simulink model "Proj3_PMSM_ForStudent"  (Simulink 8.0)
settings: Solver=ode45  StartTime=0.0  StopTime=0.5  MaxStep=1e-5  RelTol=1e-3
InitFcn:
  | Idc=0;
  | Vabc=0;
  | Iw=0;
values from neighbouring files (symbols this model uses):
  Flux = 0.7213*BaseFlux    [MSE452_Lab3_parameters.m]
  Ld = 0.7029*Lb    [MSE452_Lab3_parameters.m]
  Lq = 0.7029*Lb    [MSE452_Lab3_parameters.m]
  OMEGAb_r = OMEGAb/Ppairs    (= 41.885284054)    [MSE452_Lab3_parameters.m]
  Ppairs = 8    [MSE452_Lab3_parameters.m]
  Rs = 0.00517*Zb    [MSE452_Lab3_parameters.m]
undefined symbols (not defined in the file or in its folder): Ts
libraries: powerlib x1
settings Model: Creator=Administrator  LastModifiedBy=dw  BufferReuse=off
settings SolverCC: ZeroCrossControl=DisableAll
settings DataIOCC: SignalLoggingSaveFormat=ModelDataLogs
settings OptimizationCC: BlockReduction=off  InlineParams=on  BufferReuse=off  InitFltsAndDblsToZero=on
settings DebuggingCC: SaveWithParameterizedLinksMsg=none  SignalResolutionControl=TryResolveAllWithWarning  MultiTaskDSMMsg=warning  MultiTaskCondExecSysMsg=none  FcnCallInpInsideContextMsg=UseLocalSettings  StrictBusMsg=Warning
settings RTWCC: IncludeERTFirstTime=on
settings GRTTargetCC: TargetFcnLib=ansi_tfl_tmw.mat  CombineOutputUpdateFcns=off  GRTInterface=on

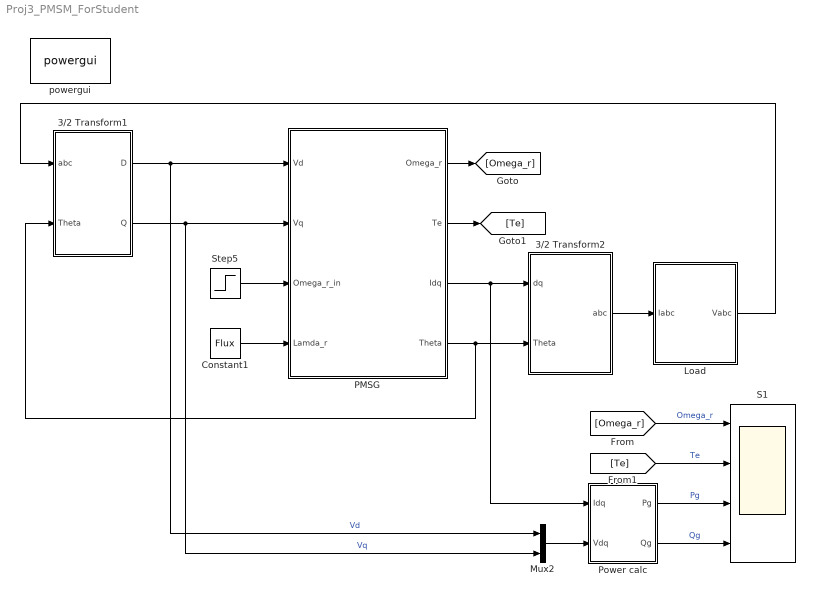
== system Proj3_PMSM_ForStudent ==
  3/2 Transform1 : Subsystem
  3/2 Transform2 : Subsystem
  Constant1 : Constant  Value=Flux
  Load : Subsystem
  Mux2 : Mux  Inputs=2
  PMSG : Subsystem
  Power calc : Subsystem
  S1 : Scope  NumInputPorts=4
      settings: TimeRange=1  YMin=-500~-30~120~1750  YMax=3500~50~210~3500  SaveName=SpeedTorquePower
  Step5 : Step  Time=0  After=1.0*OMEGAb_r  SampleTime=0
  powergui : powerlib/powergui  SimulationMode=Continuous  SolverType=Tustin  SampleTime=Ts  frequency=60  SPID=off  DisableSnubberDevices=off  DisableRonSwitches=off  DisableVfSwitches=off  SwTol=0  Interpol=off  DisplayEquations=off  FunctionMessages=off  frequencyindice=1  Pbase=100e6  ErrMax=1e-4  Iterations=50  UnitsV=kV  UnitsW=MW  echomessages=off  HookPort=off  EnableUseOfTLC=off  x0status=blocks  RestoreLinks=warning  ResistiveCurrentMeasurement=off  Frange=[0:2:500]  Ylog=off  Xlog=on  ShowGrid=off  save=off  variable=ZData  structure=GridVIWave  ZoomFFT=off  StartTime=2  cycles=12  DisplayStyle=1  fundamental=60  FreqAxis=on  MaxFrequency=60*15  frequencyindicesteady=1  RmsSteady=1  display=off  Ts=0  methode=off
  wires:
  PMSG/3(Idq) -> 3/2 Transform2/1(dq), Power calc/1(Idq)
  3/2 Transform1/2(Q) -> PMSG/2(Vq), Mux2/2  "Vq"
  3/2 Transform1/1(D) -> PMSG/1(Vd), Mux2/1  "Vd"
  PMSG/1(Omega_r) -> [Omega_r]
  PMSG/2(Te) -> [Te]
  Step5/1 -> PMSG/3(Omega_r_in)
  PMSG/4(Theta) -> 3/2 Transform2/2(Theta), 3/2 Transform1/2(Theta)
  Mux2/1 -> Power calc/2(Vdq)
  Constant1/1 -> PMSG/4(Lamda_r)
  3/2 Transform2/1(abc) -> Load/1(Iabc)
  Load/1(Vabc) -> 3/2 Transform1/1(abc)
  Power calc/2(Qg) -> S1/4  "Qg"
  Power calc/1(Pg) -> S1/3  "Pg"
  [Omega_r] -> S1/1  "Omega_r"
  [Te] -> S1/2  "Te"

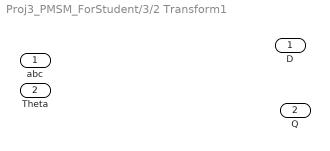
== system Proj3_PMSM_ForStudent/3/2 Transform1 ==
  abc : Inport
  Theta : Inport  Port=2
  D : Outport
  Q : Outport  Port=2

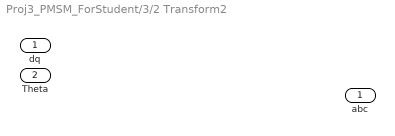
== system Proj3_PMSM_ForStudent/3/2 Transform2 ==
  dq : Inport
  Theta : Inport  Port=2
  abc : Outport

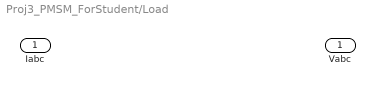
== system Proj3_PMSM_ForStudent/Load ==
  Iabc : Inport
  Vabc : Outport

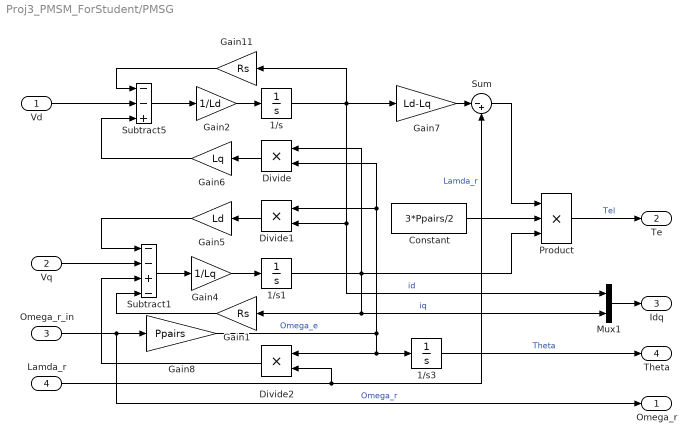
== system Proj3_PMSM_ForStudent/PMSG ==
  Vd : Inport
  Vq : Inport  Port=2
  Omega_r_in : Inport  Port=3
  Lamda_r : Inport  Port=4
  1/s : Integrator
  1/s1 : Integrator
  1/s3 : Integrator
  Constant : Constant  Value=3*Ppairs/2
  Divide : Product  Inputs=**
  Divide1 : Product  Inputs=**
  Divide2 : Product  Inputs=**
  Gain1 : Gain  Gain=Rs
  Gain11 : Gain  Gain=Rs
  Gain2 : Gain  Gain=1/Ld
  Gain4 : Gain  Gain=1/Lq
  Gain5 : Gain  Gain=Ld
  Gain6 : Gain  Gain=Lq
  Gain7 : Gain  Gain=Ld-Lq
  Gain8 : Gain  Gain=Ppairs
  Mux1 : Mux  Inputs=2
  Product : Product  Inputs=3  RndMeth=Zero
  Subtract1 : Sum  Inputs=--+-
  Subtract5 : Sum  Inputs=--+
  Sum : Sum  Inputs=|-+
  Omega_r : Outport
  Te : Outport  Port=2
  Idq : Outport  Port=3
  Theta : Outport  Port=4
  wires:
  Divide2/1 -> Subtract1/3
  Product/1 -> Te/1  "Tel"
  Constant/1 -> Product/2
  Sum/1 -> Product/1
  Gain7/1 -> Sum/1
  Gain5/1 -> Subtract1/1
  Gain6/1 -> Subtract5/3
  Divide1/1 -> Gain5/1
  Divide/1 -> Gain6/1
  1/s1/1 -> Divide/1, Product/3, Mux1/2, Gain1/1  "iq"
  Gain4/1 -> 1/s1/1
  Subtract1/1 -> Gain4/1
  1/s/1 -> Divide1/2, Mux1/1, Gain7/1, Gain11/1  "id"
  Gain2/1 -> 1/s/1
  Subtract5/1 -> Gain2/1
  Vd/1 -> Subtract5/2
  Vq/1 -> Subtract1/2
  Mux1/1 -> Idq/1
  Gain11/1 -> Subtract5/1
  Lamda_r/1 -> Divide2/2, Sum/2  "Lamda_r"
  Omega_r_in/1 -> Gain8/1, Omega_r/1  "Omega_r"
  1/s3/1 -> Theta/1  "Theta"
  Gain1/1 -> Subtract1/4
  Gain8/1 -> Divide1/1, Divide/2, Divide2/1, 1/s3/1  "Omega_e"

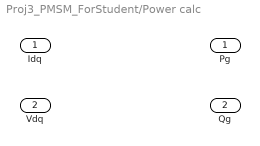
== system Proj3_PMSM_ForStudent/Power calc ==
  Idq : Inport
  Vdq : Inport  Port=2
  Pg : Outport
  Qg : Outport  Port=2
